simulink model "Continuous_to_discrete_tank_model"  (Simulink 7.6)
settings: Solver=ode45  StartTime=0.0  StopTime=10.0  RelTol=1e-3
Description:
  | Lecture 3. Continuous to discrete system representation (A,B,C,D)->(Phi,Gamma,C,D)
  | 
  | We consider state space model given by Eq.2.39-2.40 (course material)
  | with (a=-1/10,b=1/10,c=1,d=1).
  | 
  | We construct the sampled system analog. It can be demonstrated that the choice of
  | the sampling time determines the accuracy among continuous model (plant) and
  | discrete representation (model) of the plant.
  | 
  | Task 1. For the sampling time T=0.5, open the Sampler box and enter T=0.5 (sampling time)
  | Also, NEED TO CHANGE PARAMETERS OF DISCRETE STATE-SPACE module, open the module
  | and enter  for A=expm(-1/10*(T)), B=(-1/10)*(expm((-1/10)*(T))-1)*1/10, C=1 D=1. These expressions
  | are given by Eq.2.51-2.52.
  | 
  | Task 2. Repeat the same procedure for  1)  T=0.01 (observe that error is almost zero)
  |                                                               2) T=3/4pi (error increases as model accuracy decreasse due to the large sampling time)
settings Model: Creator=administrator  LastModifiedBy=administrator

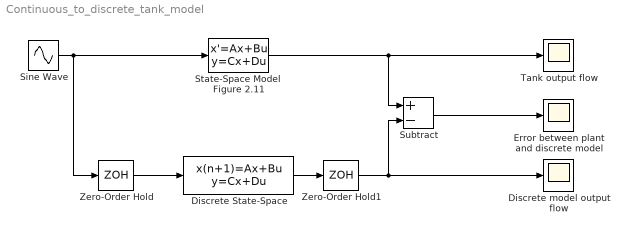
== system Continuous_to_discrete_tank_model ==
  Discrete State-Space : DiscreteStateSpace  A=expm(-1/10*(0.1))  B=(-1/10)*(expm((-1/10)*(0.1))-1)*1/10  C=1/1  SampleTime=-1
  "Discrete model output flow " : Scope
      settings: TimeRange=10  SaveName=ScopeData2
  Error between plant and discrete model : Scope
      settings: TimeRange=10
  Sine Wave : Sin  SampleTime=0
  State-Space Model  Figure 2.11 : StateSpace  A=-1/10  B=1/10  ContinuousStateAttributes='height'
  Subtract : Sum  Inputs=+-
  Tank output flow : Scope
      settings: TimeRange=10
  Zero-Order Hold : ZeroOrderHold  SampleTime=0.5
  Zero-Order Hold1 : ZeroOrderHold  SampleTime=0.01
  wires:
  Sine Wave/1 -> State-Space Model  Figure 2.11/1, Zero-Order Hold/1
  State-Space Model  Figure 2.11/1 -> Tank output flow/1, Subtract/1
  Zero-Order Hold/1 -> Discrete State-Space/1
  Discrete State-Space/1 -> Zero-Order Hold1/1
  Zero-Order Hold1/1 -> Subtract/2, "Discrete model output flow "/1
  Subtract/1 -> Error between plant and discrete model/1
